simulink model "FinalProject"  (R2022a)
settings: Solver=FixedStepAuto  StartTime=0.0  StopTime=inf  FixedStep=0.1  RelTol=1e-3
model workspace (MAT data in the model file):
  SL_ROS_VariableLengthArrays_MaxSizes.CommonInfo.ArrayTruncateAction = 'EmitWarning'
  SL_ROS_VariableLengthArrays_MaxSizes.MsgTypeMap = containers.Map
  SL_ROS_VariableLengthArrays_MaxSizes.MsgTypeMap.serialization.keys = {'sensor_msgs/Image'}
  SL_ROS_VariableLengthArrays_MaxSizes.MsgTypeMap.serialization.values{1}(1).PropertyName = 'Data'
  SL_ROS_VariableLengthArrays_MaxSizes.MsgTypeMap.serialization.values{1}(1).DataType = 'uint8'
  SL_ROS_VariableLengthArrays_MaxSizes.MsgTypeMap.serialization.values{1}(1).MaxLength = 921600
  SL_ROS_VariableLengthArrays_MaxSizes.MsgTypeMap.serialization.values{1}(2).PropertyName = 'Encoding'
  SL_ROS_VariableLengthArrays_MaxSizes.MsgTypeMap.serialization.values{1}(2).DataType = 'uint8'
  SL_ROS_VariableLengthArrays_MaxSizes.MsgTypeMap.serialization.values{1}(2).MaxLength = 128
  SL_ROS_VariableLengthArrays_MaxSizes.MsgTypeMap.serialization.uniformity = 0
  SL_ROS_VariableLengthArrays_MaxSizes.MsgTypeMap.serialization.keyType = 'char'
  SL_ROS_VariableLengthArrays_MaxSizes.MsgTypeMap.serialization.valueType = 'any'
values from neighbouring files (symbols this model uses):
  WList = [0, 0, 0 ... (first row only)    [A1_WayAndObj.m]    (also in A1_WayDefAndObjSpawn.m; WList.mat = [0 6 3 9 12 15 18 0 0 6 9 0 ... (21 elements, 7x3)])
undefined symbols (not defined in the file or in its folder): Angular, gray, Linear, Rec, SDTV
libraries: robotlib x7, simulink x3, visiontextngfix x2, visionstatistics x2, visionconversions x1
settings Model: Creator=jacopo  LastModifiedBy=jacopo
settings OptimizationCC: EnhancedBackFolding=on  PassReuseOutputArgsAs=Individual arguments  ZeroExternalMemoryAtStartup=off  ZeroInternalMemoryAtStartup=off  MaxStackSize=64  OptimizeBlockOrder=speed  DifferentSizesBufferReuse=on  OptimizationCustomize=off  EfficientTunableParamExpr=on
settings DebuggingCC: ParameterTunabilityLossMsg=error
settings HardwareCC: ProdBitPerPointer=32  ProdBitPerSizeT=32  ProdBitPerPtrDiffT=32  ProdLargestAtomicFloat=None  ProdIntDivRoundTo=Undefined  ProdEndianess=Unspecified  ProdWordSize=32  ProdHWDeviceType=Generic->Unspecified (assume 32-bit Generic)
settings SFSimCC: MATLABDynamicMemAlloc=off
settings RTWCC: SystemTargetFile=ert.tlc  HardwareBoard=Robot Operating System (ROS)  TLCOptions="-aInlineSetEventsForThisBaseRateFcn=TLC_FALSE -aSuppressMultiTaskScheduler=TLC_FALSE  -aRateBasedStepFcn=0"  TemplateMakefile=ert_default_tmf  Toolchain=Catkin  TargetLang=C++
settings CodeAppCC: ForceParamTrailComments=on  IgnoreCustomStorageClasses=off  OperatorAnnotations=on  SimulinkDataObjDesc=on  SFDataObjDesc=on  InsertBlockDesc=on

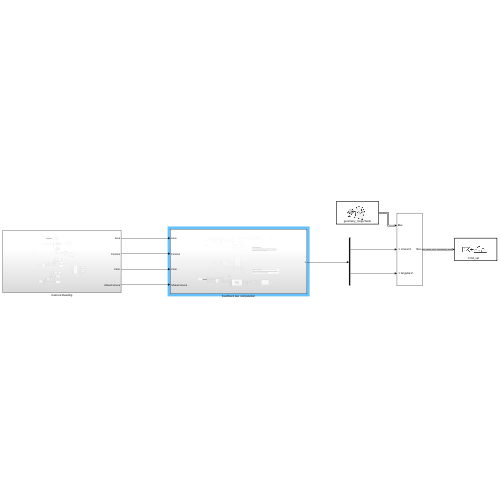
[thumbnail: Simulink's stored preview of the top-level diagram]
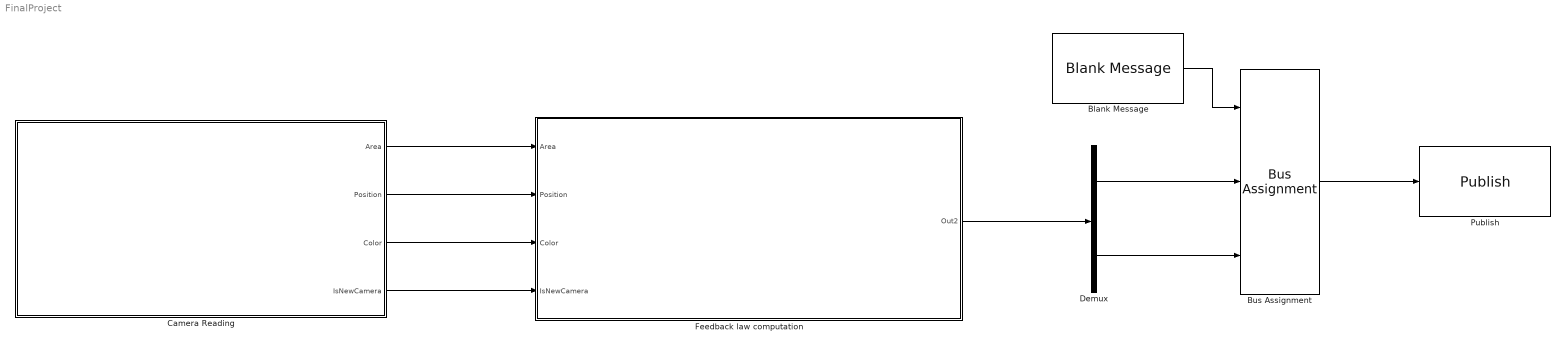
== system FinalProject ==
  Blank Message : robotlib/Blank Message  messageClass=Message  entityType=geometry_msgs/Twist  messageType=geometry_msgs/Twist  SampleTime=inf  legacyBusStruct=off
  Bus Assignment : BusAssignment  AssignedSignals=Linear.X,Angular.Z
  Camera Reading : Subsystem
  Demux : Demux  Outputs=2
  Feedback law computation : Subsystem
  Publish : robotlib/Publish  topicSource=Select from ROS network  topic=/cmd_vel  messageType=geometry_msgs/Twist  legacyBusStruct=off  messageQueueLength=1
  wires:
  Demux/1 -> Bus Assignment/2
  Blank Message/1 -> Bus Assignment/1
  Demux/2 -> Bus Assignment/3
  Bus Assignment/1 -> Publish/1
  Feedback law computation/1(Out2) -> Demux/1
  Camera Reading/4(IsNewCamera) -> Feedback law computation/4(IsNewCamera)
  Camera Reading/3(Color) -> Feedback law computation/3(Color)
  Camera Reading/2(Position) -> Feedback law computation/2(Position)
  Camera Reading/1(Area) -> Feedback law computation/1(Area)

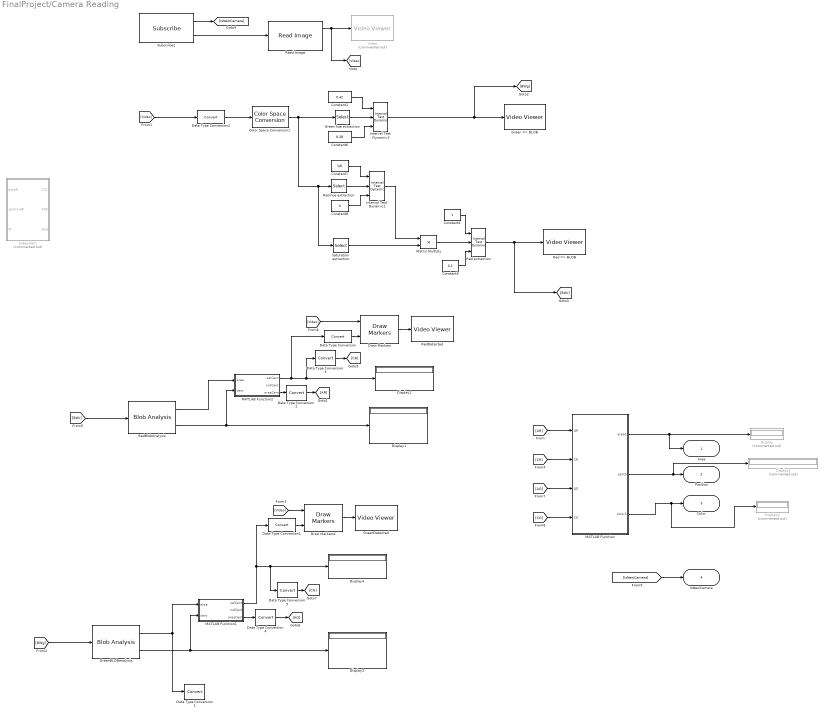
== system FinalProject/Camera Reading ==
  Color Space Conversion1 : visionconversions/Color Space  Conversion  conversion=Obsolete  conversionActive=R'G'B' to HSV  wp_str=D65  rec=Rec. 601 (SDTV)  sys=1125/60/2:1  imagePorts=One multidimensional signal
  Constant1 : Constant  Value=0.42
  Constant4 : Constant
  Constant5 : Constant  Value=0.1
  Constant6 : Constant  Value=0.28
  Constant7 : Constant  Value=1/6
  Constant8 : Constant  Value=0
  Data Type Conversion{,1,1..2,2..5} (8 alike) : DataTypeConversion  SaturateOnIntegerOverflow=off  RndMeth=Floor
  Display : Display  Commented=on
  Display{1..4} (4 alike) : Display
  Display5 : Display  Commented=on
  Display6 : Display  Commented=on
  Draw Markers : visiontextngfix/Draw Markers  shape=Star  size=30  fill=off  fillClrSource=Specify via dialog  display=User-specified value  intensity=200  color=[255 0 0]  opacity=0.6  viewport=Entire image  antialiasing=off  inType=Obsolete  imagePorts=One multidimensional signal  roundingMode=Floor  overflowMode=off  memoryMode=Specify word length  memoryWordLength=16  memoryFracLength=15  prodOutputMode=Binary point scaling  prodOutputWordLength=32  prodOutputFracLength=14
      settings: SourceProductBaseCode=VP
  Draw Markers1 : visiontextngfix/Draw Markers  shape=Plus  size=30  fill=off  fillClrSource=Specify via dialog  display=User-specified value  intensity=200  color=[255 0 0]  opacity=0.6  viewport=Entire image  antialiasing=off  inType=Obsolete  imagePorts=One multidimensional signal  roundingMode=Floor  overflowMode=off  memoryMode=Specify word length  memoryWordLength=16  memoryFracLength=15  prodOutputMode=Binary point scaling  prodOutputWordLength=32  prodOutputFracLength=14
      settings: SourceProductBaseCode=VP
  Green => BLOB : VideoViewer  colormapValue=gray(256)  FigPos=[963 1078 601 330]
  Green hue extraction : Selector  NumberOfDimensions=3  InputPortWidth=3  IndexOptions=Index vector (dialog),Index vector (dialog),Index vector (dialog)  Indices=[1:480],[1:640],1  OutputSizes=1,1,1
  GreenBLOBanalysis : visionstatistics/Blob Analysis  Tag=vipblks_row_conv  area=on  centroid=on  bBox=off  majorAxis=off  minorAxis=off  angle=off  eccentricity=off  equivDiameterSq=off  extent=off  perimeter=off  outDT=double  conn=8  isLabel=off  maxBlobs=3  warnIfNumBlobsExceeded=on  isCount=off  useMinArea=off  minArea=0  useMaxArea=off  maxArea=intmax('uint32')  excludeBorderBlob=off  isOutVarDim=off  isFill=on  fillValues=-1  roundingMode=Floor  overflowMode=off  prodOutputMode=Binary point scaling  prodOutputWordLength=32  prodOutputFracLength=16  accumMode=Binary point scaling  accumWordLength=32  accumFracLength=0  outputMode=Binary point scaling  outputWordLength=32  outputFracLength=16  firstCoeffMode=Binary point scaling  firstCoeffWordLength=16  firstCoeffFracLength=14  secondCoeffMode=Binary point scaling  secondCoeffWordLength=32  secondCoeffFracLength=16
  GreenDetected : VideoViewer  colormapValue=gray(256)  FigPos=[253 580 593 356]
  Interval Test Dynamic1 : simulink/Logic and Bit Operations/Interval Test Dynamic  IntervalClosedRight=on  IntervalClosedLeft=on  OutDataTypeStr=boolean
      settings: SourceProductBaseCode=SL
  Interval Test Dynamic3 : simulink/Logic and Bit Operations/Interval Test Dynamic  IntervalClosedRight=on  IntervalClosedLeft=on  OutDataTypeStr=boolean
      settings: SourceProductBaseCode=SL
  MATLAB Function : MATLAB Function  TreatAsAtomicUnit=on
  MATLAB Function1 : MATLAB Function  TreatAsAtomicUnit=on
  MATLAB Function2 : MATLAB Function  TreatAsAtomicUnit=on
  Matrix Multiply : Product
  Read Image : robotlib/Read Image  MaximumImageSize=[480, 640]  ImageEncoding=rgb8  ShowAlphaOutput=off  ShowErrorCodeOutput=on  VariableSizeOutputs=off
      settings: SourceProductBaseCode=RR
  Red => BLOB : VideoViewer  colormapValue=gray(256)  FigPos=[650 1078 581 344]
  Red extraction : simulink/Logic and Bit Operations/Interval Test Dynamic  IntervalClosedRight=on  IntervalClosedLeft=on  OutDataTypeStr=boolean
      settings: SourceProductBaseCode=SL
  Red hue extraction : Selector  NumberOfDimensions=3  InputPortWidth=3  IndexOptions=Index vector (dialog),Index vector (dialog),Index vector (dialog)  Indices=[1:480],[1:640],1  OutputSizes=1,1,1
  RedBlobAnalysis : visionstatistics/Blob Analysis  Tag=vipblks_row_conv  area=on  centroid=on  bBox=off  majorAxis=off  minorAxis=off  angle=off  eccentricity=off  equivDiameterSq=off  extent=off  perimeter=off  outDT=double  conn=8  isLabel=off  maxBlobs=3  warnIfNumBlobsExceeded=on  isCount=off  useMinArea=off  minArea=0  useMaxArea=off  maxArea=intmax('uint32')  excludeBorderBlob=off  isOutVarDim=off  isFill=on  fillValues=-1  roundingMode=Floor  overflowMode=off  prodOutputMode=Binary point scaling  prodOutputWordLength=32  prodOutputFracLength=16  accumMode=Binary point scaling  accumWordLength=32  accumFracLength=0  outputMode=Binary point scaling  outputWordLength=32  outputFracLength=16  firstCoeffMode=Binary point scaling  firstCoeffWordLength=16  firstCoeffFracLength=14  secondCoeffMode=Binary point scaling  secondCoeffWordLength=32  secondCoeffFracLength=16
  RedDetected : VideoViewer  colormapValue=gray(256)  FigPos=[255 1064 583 363]
  Saturation extraction : Selector  NumberOfDimensions=3  InputPortWidth=3  IndexOptions=Index vector (dialog),Index vector (dialog),Index vector (dialog)  Indices=[1:480],[1:640],2  OutputSizes=1,1,1
  Subscribe1 : robotlib/Subscribe  topicSource=Select from ROS network  topic=/camera/rgb/image_raw  messageType=sensor_msgs/Image  SampleTime=-1  legacyBusStruct=off  messageQueueLength=1
  Subsystem : Subsystem  Commented=on
  Video : VideoViewer  Commented=on  colormapValue=gray(256)  FigPos=[689 794 566 352]
  Area : Outport
  Position : Outport  Port=2
  Color : Outport  Port=3
  IsNewCamera : Outport  Port=4
  wires:
  Subscribe1/2 -> Read Image/1
  Constant7/1 -> Interval Test Dynamic1/1
  Read Image/1 -> [Video], Video/1
  Saturation extraction/1 -> Matrix Multiply/2
  Color Space Conversion1/1 -> Green hue extraction/1, Saturation extraction/1, Red hue extraction/1
  [Video] -> Data Type Conversion2/1
  Subscribe1/1 -> [IsNewCamera]
  Constant4/1 -> Red extraction/1
  Constant5/1 -> Red extraction/3
  Red hue extraction/1 -> Interval Test Dynamic1/2
  Red extraction/1 -> [BWr], Red => BLOB/1
  Matrix Multiply/1 -> Red extraction/2
  Interval Test Dynamic1/1 -> Matrix Multiply/1
  Constant8/1 -> Interval Test Dynamic1/3
  Data Type Conversion2/1 -> Color Space Conversion1/1
  Green hue extraction/1 -> Interval Test Dynamic3/2
  Constant6/1 -> Interval Test Dynamic3/3
  Constant1/1 -> Interval Test Dynamic3/1
  Interval Test Dynamic3/1 -> [BWg], Green => BLOB/1
  [BWr] -> RedBlobAnalysis/1
  RedBlobAnalysis/2 -> Display1/1, MATLAB Function2/2(cent)
  Draw Markers/1 -> RedDetected/1
  Data Type Conversion/1 -> Draw Markers/2
  [Video] -> Draw Markers/1
  RedBlobAnalysis/1 -> MATLAB Function2/1(area)
  MATLAB Function2/1(selCent) -> Data Type Conversion3/1, Display2/1, Data Type Conversion/1
  GreenBLOBanalysis/1 -> MATLAB Function1/1(area), Data Type Conversion1/1
  MATLAB Function1/1(selCent) -> Data Type Conversion1/1, Data Type Conversion5/1, Display4/1
  [Video] -> Draw Markers1/1
  Data Type Conversion1/1 -> Draw Markers1/2
  Draw Markers1/1 -> GreenDetected/1
  GreenBLOBanalysis/2 -> Display3/1, MATLAB Function1/2(cent)
  [BWg] -> GreenBLOBanalysis/1
  MATLAB Function/2(centS) -> Display5/1, Position/1
  MATLAB Function/3(colorS) -> Display6/1, Color/1
  [AR] -> MATLAB Function/1(AR)
  [CR] -> MATLAB Function/2(CR)
  [AG] -> MATLAB Function/3(AG)
  [CG] -> MATLAB Function/4(CG)
  MATLAB Function2/3(areaCent) -> Data Type Conversion2/1
  Data Type Conversion2/1 -> [AR]
  Data Type Conversion3/1 -> [CR]
  MATLAB Function1/3(areaCent) -> Data Type Conversion4/1
  Data Type Conversion4/1 -> [AG]
  Data Type Conversion5/1 -> [CG]
  MATLAB Function/1(areaS) -> Display/1, Area/1
  [IsNewCamera] -> IsNewCamera/1

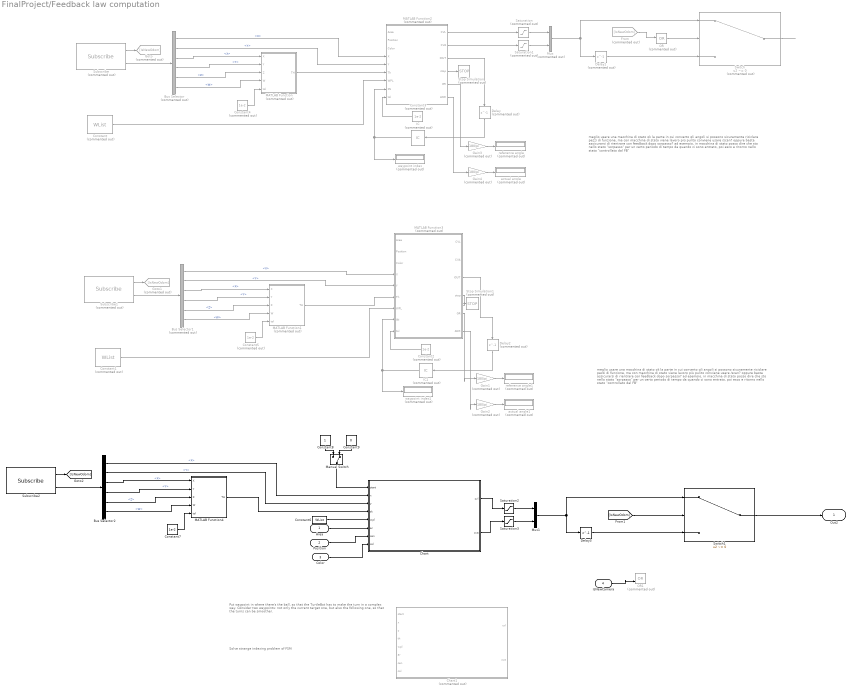
== system FinalProject/Feedback law computation ==
  note: Solve strange indexing problem of FSM
  note: Put waypoint in where there's the ball, so that the TurtleBot has to make the turn in a complex way.
      | Consider two waypoints: not only the current target one, but also the following one, so that the turns can be smoother.
  note: meglio usare una macchina di stato
      | ok la parte in cui converto gli angoli
      | si possono sicuramente riciclare pezzi di funzione, ma con macchina di stato viene lavoro più pulito
      |
      | conviene usare /scan? oppure basta assicurarsi di rientrare con feedback dopo sorpasso? ad esempio, in macchina di stato posso dire che sto nello stato "sorpasso" per un certo periodo di tempo da quando ci sono entrato, poi esco e ritorno nello stato "controllato dal FB"
  note: meglio usare una macchina di stato
      | ok la parte in cui converto gli angoli
      | si possono sicuramente riciclare pezzi di funzione, ma con macchina di stato viene lavoro più pulito
      |
      | conviene usare /scan? oppure basta assicurarsi di rientrare con feedback dopo sorpasso? ad esempio, in macchina di stato posso dire che sto nello stato "sorpasso" per un certo periodo di tempo da quando ci sono entrato, poi esco e ritorno nello stato "controllato dal FB"
  Area : Inport
  Position : Inport  Port=2
  Color : Inport  Port=3
  IsNewCamera : Inport  Port=4
  Bus Selector : BusSelector  Commented=on  OutputSignals=Pose.Pose.Position.X,Pose.Pose.Position.Y,Pose.Pose.Orientation.X,Pose.Pose.Orientation.Y,Pose.Pose.Orientation.Z,Pose.Pose.Orientation.W
  Bus Selector1 : BusSelector  Commented=on  OutputSignals=Pose.Pose.Position.X,Pose.Pose.Position.Y,Pose.Pose.Orientation.X,Pose.Pose.Orientation.Y,Pose.Pose.Orientation.Z,Pose.Pose.Orientation.W
  Bus Selector2 : BusSelector  OutputSignals=Pose.Pose.Position.X,Pose.Pose.Position.Y,Pose.Pose.Orientation.X,Pose.Pose.Orientation.Y,Pose.Pose.Orientation.Z,Pose.Pose.Orientation.W
  Chart : Stateflow chart  TreatAsAtomicUnit=on
  Chart1 : Stateflow chart  Commented=on  TreatAsAtomicUnit=on
  Constant : Constant  Commented=on  Value=WList
  Constant1 : Constant  Commented=on  Value=WList
  Constant{2..5} (4 alike) : Constant  Commented=on  Value=1e-2
  Constant6 : Constant  Value=WList
  Constant7 : Constant  Value=1e-2
  Constant8 : Constant
  Constant9 : Constant  Value=0
  Delay : Delay  Commented=on  DelayLength=1
  Delay1 : Delay  Commented=on  DelayLength=1
  Delay2 : Delay  Commented=on  DelayLength=1
  Delay3 : Delay  DelayLength=1
  From : From  Commented=on  GotoTag=IsNewOdom
  Gain{1..4} (4 alike) : Gain  Commented=on  Gain=180/pi
  Goto : Goto  Commented=on  GotoTag=IsNewOdom
  Goto1 : Goto  Commented=on  GotoTag=IsNewOdom
  IC : InitialCondition  Commented=on
  IC1 : InitialCondition  Commented=on
  MATLAB Function : MATLAB Function  Commented=on  TreatAsAtomicUnit=on
  MATLAB Function1 : MATLAB Function  Commented=on  TreatAsAtomicUnit=on
  MATLAB Function2 : MATLAB Function  Commented=on  TreatAsAtomicUnit=on
  MATLAB Function3 : MATLAB Function  Commented=on  TreatAsAtomicUnit=on
  MATLAB Function4 : MATLAB Function  TreatAsAtomicUnit=on
  Manual Switch : ManualSwitch  CurrentSetting=0
  Mux : Mux  Commented=on  Inputs=2
  Mux1 : Mux  Inputs=2
  OR : Logic  Commented=on  Operator=OR  IconShape=distinctive  AllPortsSameDT=off  OutDataTypeStr=boolean
  OR1 : Logic  Commented=on  Operator=OR  IconShape=distinctive  AllPortsSameDT=off  OutDataTypeStr=boolean
  Saturation : Saturate  Commented=on  UpperLimit=0.2  LowerLimit=-0.2
  Saturation1 : Saturate  Commented=on  UpperLimit=0.4  LowerLimit=-0.4
  Saturation2 : Saturate  UpperLimit=0.2  LowerLimit=-0.2
  Saturation3 : Saturate  UpperLimit=0.4  LowerLimit=-0.4
  Stop Simulation : Stop  Commented=on
  Stop Simulation1 : Stop  Commented=on
  Subscribe : robotlib/Subscribe  Commented=on  topicSource=Select from ROS network  topic=/odom  messageType=nav_msgs/Odometry  SampleTime=-1  legacyBusStruct=off  messageQueueLength=1
  Subscribe1 : robotlib/Subscribe  Commented=on  topicSource=Select from ROS network  topic=/odom  messageType=nav_msgs/Odometry  SampleTime=-1  legacyBusStruct=off  messageQueueLength=1
  Subscribe2 : robotlib/Subscribe  topicSource=Select from ROS network  topic=/odom  messageType=nav_msgs/Odometry  SampleTime=-1  legacyBusStruct=off  messageQueueLength=1
  Switch : Switch  Commented=on  Criteria=u2 ~= 0  SaturateOnIntegerOverflow=off  InputSameDT=off
  Switch1 : Switch  Criteria=u2 ~= 0  SaturateOnIntegerOverflow=off  InputSameDT=off
  actual angle : Display  Commented=on
  actual angle1 : Display  Commented=on
  reference angle : Display  Commented=on
  reference angle1 : Display  Commented=on
  waypoint index : Display  Commented=on
  waypoint index1 : Display  Commented=on
  Out2 : Outport
  wires:
  Delay/1 -> IC/1
  IC/1 -> MATLAB Function2/8(IIN), waypoint index/1
  Constant/1 -> MATLAB Function2/7(WPL)
  Constant3/1 -> MATLAB Function2/9(tol)
  Bus Selector/6 -> MATLAB Function/4(W)  "<W>"
  Gain4/1 -> actual angle/1
  MATLAB Function2/4(stop) -> Stop Simulation/1
  Bus Selector/5 -> MATLAB Function/3(Z)  "<Z>"
  MATLAB Function2/6(ANG) -> Gain4/1
  Bus Selector/3 -> MATLAB Function/1(X)  "<X>"
  Saturation/1 -> Mux/1
  MATLAB Function/1(TH) -> MATLAB Function2/6(Th)
  MATLAB Function2/5(GR) -> Gain3/1
  Gain3/1 -> reference angle/1
  MATLAB Function2/2(CVA) -> Saturation1/1
  MATLAB Function2/1(CVL) -> Saturation/1
  MATLAB Function2/3(IOUT) -> Delay/1
  Subscribe/1 -> Goto/1
  Subscribe/2 -> Bus Selector/1
  Constant4/1 -> MATLAB Function/5(tol)
  Bus Selector/2 -> MATLAB Function2/5(Y)  "<Y>"
  Bus Selector/1 -> MATLAB Function2/4(X)  "<X>"
  Saturation1/1 -> Mux/2
  Bus Selector/4 -> MATLAB Function/2(Y)  "<Y>"
  From/1 -> OR/1
  Delay1/1 -> Switch/3
  Mux/1 -> Switch/1, Delay1/1
  Switch/1 -> ?
  OR/1 -> Switch/2
  ? -> OR/2
  MATLAB Function3/3(IOUT) -> Delay2/1
  Bus Selector1/1 -> MATLAB Function3/4(X)  "<X>"
  Constant2/1 -> MATLAB Function3/9(tol)
  Gain2/1 -> actual angle1/1
  MATLAB Function3/5(GR) -> Gain1/1
  IC1/1 -> MATLAB Function3/8(IIN), waypoint index1/1
  Gain1/1 -> reference angle1/1
  Constant1/1 -> MATLAB Function3/7(WPL)
  MATLAB Function3/6(ANG) -> Gain2/1
  Bus Selector1/6 -> MATLAB Function1/4(W)  "<W>"
  MATLAB Function3/4(stop) -> Stop Simulation1/1
  MATLAB Function1/1(TH) -> MATLAB Function3/6(Th)
  Bus Selector1/5 -> MATLAB Function1/3(Z)  "<Z>"
  Subscribe1/2 -> Bus Selector1/1
  Bus Selector1/2 -> MATLAB Function3/5(Y)  "<Y>"
  Subscribe1/1 -> Goto1/1
  Delay2/1 -> IC1/1
  Constant5/1 -> MATLAB Function1/5(tol)
  Bus Selector1/3 -> MATLAB Function1/1(X)  "<X>"
  Bus Selector1/4 -> MATLAB Function1/2(Y)  "<Y>"
  Color/1 -> Chart/8(col)
  Position/1 -> Chart/7(cen)
  Area/1 -> Chart/6(ar)
  Constant6/1 -> Chart/5(wpl)
  Bus Selector2/1 -> Chart/2(x)  "<X>"
  Constant7/1 -> MATLAB Function4/5(tol)
  Bus Selector2/6 -> MATLAB Function4/4(W)  "<W>"
  MATLAB Function4/1(TH) -> Chart/4(th)
  Bus Selector2/5 -> MATLAB Function4/3(Z)  "<Z>"
  Subscribe2/1 -> [IsNewOdom]
  Bus Selector2/3 -> MATLAB Function4/1(X)  "<X>"
  Subscribe2/2 -> Bus Selector2/1
  Bus Selector2/2 -> Chart/3(y)  "<Y>"
  Bus Selector2/4 -> MATLAB Function4/2(Y)  "<Y>"
  Manual Switch/1 -> Chart/1(start)
  Constant8/1 -> Manual Switch/1
  Constant9/1 -> Manual Switch/2
  Saturation2/1 -> Mux1/1
  Switch1/1 -> Out2/1
  Chart/2(cva) -> Saturation3/1
  Chart/1(cvl) -> Saturation2/1
  [IsNewOdom] -> Switch1/2
  IsNewCamera/1 -> OR1/2
  Saturation3/1 -> Mux1/2
  Mux1/1 -> Switch1/1, Delay3/1
  Delay3/1 -> Switch1/3

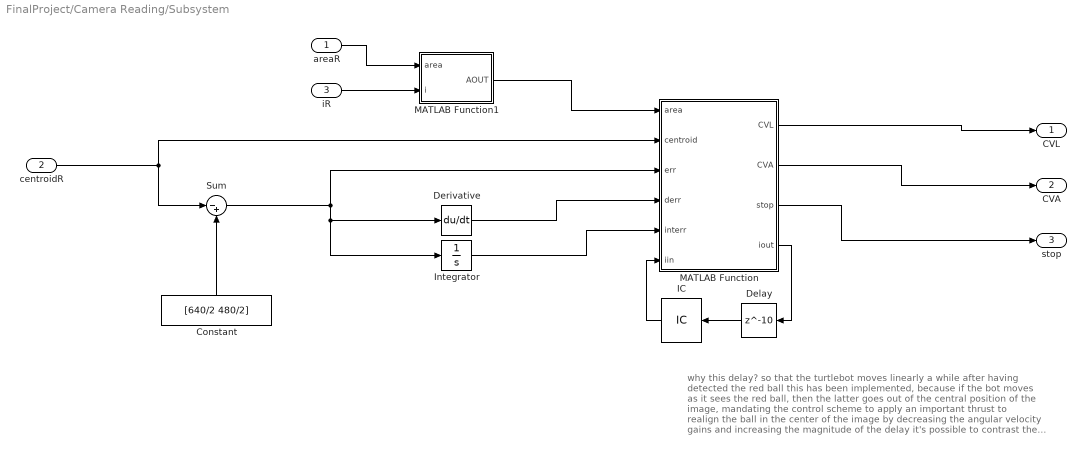
== system FinalProject/Camera Reading/Subsystem ==
  note: why this delay? so that the turtlebot moves linearly a while after
      | having detected the red ball
      | this has been implemented, because if the bot moves as it sees
      | the red ball, then the latter goes out of the central position of the image,
      | mandating the control scheme to apply an important thrust to realign
      | the ball in the center of the image
      | by decreasing the angular velocity gains and increasing the magnitude
      | of the delay it's possible to contrast the wobbly motion, caused by
      | a synergic cooperation of high gains and moving linearly too early
  areaR : Inport
  centroidR : Inport  Port=2
  iR : Inport  Port=3
  Constant : Constant  Value=[640/2 480/2]  VectorParams1D=off
  Delay : Delay  DelayLength=10
  Derivative : Derivative
  IC : InitialCondition  Value=0
  Integrator : Integrator
  MATLAB Function : MATLAB Function  TreatAsAtomicUnit=on
  MATLAB Function1 : MATLAB Function  TreatAsAtomicUnit=on
  Sum : Sum  Inputs=|-+
  CVL : Outport
  CVA : Outport  Port=2
  stop : Outport  Port=3
  wires:
  MATLAB Function/3(stop) -> stop/1
  areaR/1 -> MATLAB Function1/1(area)
  MATLAB Function/2(CVA) -> CVA/1
  MATLAB Function/1(CVL) -> CVL/1
  MATLAB Function1/1(AOUT) -> MATLAB Function/1(area)
  iR/1 -> MATLAB Function1/2(i)
  centroidR/1 -> Sum/1, MATLAB Function/2(centroid)
  Constant/1 -> Sum/2
  Sum/1 -> Integrator/1, Derivative/1, MATLAB Function/3(err)
  Derivative/1 -> MATLAB Function/4(derr)
  Integrator/1 -> MATLAB Function/5(interr)
  Delay/1 -> IC/1
  MATLAB Function/4(iout) -> Delay/1
  IC/1 -> MATLAB Function/6(iin)

== matlab function FinalProject/Camera Reading/Subsystem/MATLAB Function ==
  data: area input; CVL output; centroid input; CVA output; err input; stop output; derr input; interr input; iin input; iout output
function [CVL, CVA, stop, iout] = fcn(area, centroid, err, derr, interr, iin)

NC = 2; % max number of centroids
NoCV = - ones(NC, 2);

if centroid == NoCV
    CVL = 0;
    CVA = 0.2;
    iout = 0; %add
else
    iout = 1; %add
    kPL = 0.05;
%     kPA = 0.1;
%     kPA = 0.01;
    kPA = 0.003; % 0.01 is too high % 0.005 mmmh almost
    kDA = 0.01*0;
    kIA = 0;
    
    ERR = err(1);
    dERR = derr(1);
    intERR = interr(1);

    if iin == 1  %add
        CVL = kPL*area;
    else
        CVL = 0;
    end

    CVA = kPA*ERR + kDA*dERR + kIA*intERR;
end

maxA = 0.9*(640*480);

if area < maxA
    stop = 0;
else
    CVL = 0;
    CVA = 0;
    stop = 1;
end


% % centroidsel = centroid( centroid ~= [-1 -1])'; % not that robust

== matlab function FinalProject/Camera Reading/MATLAB Function2 ==
  data: area input; cent input; selCent output; indCent output; areaCent output
function [selCent, indCent, areaCent]  = fcn(area,cent)

[areaCent, indCent] = max(area);

if ~isempty(indCent)
    selCent = cent(indCent,:);
else 
    selCent = [0,0];
end

== matlab function FinalProject/Camera Reading/Subsystem/MATLAB Function1 ==
  data: area input; AOUT output; i input
function AOUT = fcn(area, i)

AOUT = area(i, 1);

== matlab function FinalProject/Camera Reading/MATLAB Function ==
  data: AR input; CR input; areaS output; centS output; colorS output; AG input; CG input
function [areaS, centS, colorS] = fcn(AR, CR, AG, CG)

% 1 is red, 2 is green, 0 is none

if AR > AG
    areaS = AR;
    centS = CR;
    colorS = 1;
elseif AR < AG
    areaS = AG;
    centS = CG;
    colorS = 2;
else
    areaS = 0;
    centS = [0 0];
    colorS = 0;
end

== matlab function FinalProject/Feedback law computation/MATLAB Function ==
  data: X input; TH output; Y input; Z input; W input; tol input
function TH = fromQuat2Eu(X, Y, Z, W, tol)



ANGLE = quat2eul([W, X, Y, Z]);

TH = ANGLE(1);

== matlab function FinalProject/Feedback law computation/MATLAB Function2 ==
  data: Area input; Position input; Color input; X input; CVL output; Y input; Th input; WPL input; CVA output; IOUT output; IIN input; stop output; tol input; GR output; ANG output
function [CVL, CVA, IOUT, stop, GR, ANG] = FBRegulator(Area, Position, Color, X, Y, Th, WPL, IIN, tol)

% kPL = 1;
kPA = 2; %0.8 %1.2

POSr = WPL(IIN, :);

Xr = POSr(1); Yr = POSr(2); Thr = POSr(3);

if pi < Thr && Thr < 2*pi
    Thr = Thr - 2*pi;
end

Gr = Thr;

Z = (Xr - X) + 1i*(Yr - Y);

dist = abs(Z);

% if dist <= 0.2
%     kPL = 0.4;
% end

if dist <= 0.1

    if (Th > tol) && (- pi + tol < Gr && Gr < - pi/2 - tol) % Gr < - tol
        Gr = Gr + 2*pi;
    elseif (- pi + tol < Th && Th < - pi/2 - tol) && (Gr > tol)
        Th = Th + 2*pi;
    end
    
else

    Gr = angle(Z);

    if (Th > tol) && (- pi + tol < Gr && Gr < - pi/2 - tol) % Gr < - tol
        Gr = Gr + 2*pi;
    elseif (- pi + tol < Th && Th < - pi/2 - tol) && (Gr > tol)
        Th = Th + 2*pi;
    end

end

errTh = Gr - Th;
GR = Gr;

ANG = Th;

% CVL = kPL*dist;
% CVL = kPL*0.1;
% CVL = kPL*0.2; % faster attempt
% CVL = 0.45*dist; %0.8 original, %0.4 not robust
% CVA = kPA*errTh;


if dist <= 0.05 
   stop = 0;
   CVL = 0;
   CVA = kPA*errTh;
   if abs(errTh) <= 0.05
        IOUT = IIN + 1;
        if IIN == 6
            CVA = 0;
            stop = 1;
        end
   else
       IOUT = IIN;
   end
else
    if Area > 0.2*(480*640)
        if Color == 1
            CVL = 0.15;
            CVA = 0.3;
        elseif Color == 2
            CVL = 0.15;
            CVA = -0.3;
        else
            CVA = 0.1;
            CVL = 0.1;
        end
%        a variable can be outputted with a delay, to make sure we will
%        not exit the overtake phase
    else
        CVL = 0.1*dist;
        CVA = kPA*errTh;
    end
%     CVA = kPA*errTh;
    IOUT = IIN;
    stop = 0;
end

== matlab function FinalProject/Feedback law computation/MATLAB Function1 ==
  data: X input; TH output; Y input; Z input; W input; tol input
function TH = fromQuat2Eu(X, Y, Z, W, tol)



ANGLE = quat2eul([W, X, Y, Z]);

TH = ANGLE(1);

== matlab function FinalProject/Feedback law computation/MATLAB Function3 ==
  data: Area input; Position input; Color input; X input; CVL output; Y input; Th input; WPL input; CVA output; IOUT output; IIN input; stop output; tol input; GR output; ANG output
function [CVL, CVA, IOUT, stop, GR, ANG] = FBRegulator(Area, Position, Color, X, Y, Th, WPL, IIN, tol)

% kPL = 1;
kPA = 2; %0.8 %1.2

POSr = WPL(IIN, :);

Xr = POSr(1); Yr = POSr(2); Thr = POSr(3);

if pi < Thr && Thr < 2*pi
    Thr = Thr - 2*pi;
end

Gr = Thr;

Z = (Xr - X) + 1i*(Yr - Y);

dist = abs(Z);

% if dist <= 0.2
%     kPL = 0.4;
% end

if dist <= 0.1

    if (Th > tol) && (- pi + tol < Gr && Gr < - pi/2 - tol) % Gr < - tol
        Gr = Gr + 2*pi;
    elseif (- pi + tol < Th && Th < - pi/2 - tol) && (Gr > tol)
        Th = Th + 2*pi;
    end
    
else

    Gr = angle(Z);

    if (Th > tol) && (- pi + tol < Gr && Gr < - pi/2 - tol) % Gr < - tol
        Gr = Gr + 2*pi;
    elseif (- pi + tol < Th && Th < - pi/2 - tol) && (Gr > tol)
        Th = Th + 2*pi;
    end

end

errTh = Gr - Th;
GR = Gr;

ANG = Th;

% CVL = kPL*dist;
% CVL = kPL*0.1;
% CVL = kPL*0.2; % faster attempt
% CVL = 0.45*dist; %0.8 original, %0.4 not robust
% CVA = kPA*errTh;


if dist <= 0.05 
   stop = 0;
   CVL = 0;
   CVA = kPA*errTh;
   if abs(errTh) <= 0.05
        IOUT = IIN + 1;
        if IIN == 6
            CVA = 0;
            stop = 1;
        end
   else
       IOUT = IIN;
   end
else
    if Area > 0.2*(480*640)
        if Color == 1
            CVL = 0.15;
            CVA = 0.3;
        elseif Color == 2
            CVL = 0.15;
            CVA = -0.3;
        else
            CVA = 0.1;
            CVL = 0.1;
        end
%        a variable can be outputted with a delay, to make sure we will
%        not exit the overtake phase
    else
        CVL = 0.1*dist;
        CVA = kPA*errTh;
    end
%     CVA = kPA*errTh;
    IOUT = IIN;
    stop = 0;
end

== stateflow chart FinalProject/Feedback law computation/Chart ==
  state RedOvertaking
    [cvl, cva, overT, aDec] = overtakingR(cvl, cva, overT);
  state FBMotion
    [Dist, ErrTh] = disterrfun(x, y, th, wpl, index)
    cvl = kPL*Dist;
    cva = kPA*ErrTh;
  state Still
    cvl = 0;
    cva = 0;
    index = 1;
    kPL = 0.48;
    kPA = 2;
    overT = 0;
  state GreenOvertaking
    [cvl, cva, overT, aDec] = overtakingG(cvl, cva, overT);
  state Turning
    [Dist, ErrTh] = disterrfun(x, y, th, wpl, index)
    cvl = 0;
    cva = (0.9*kPA)*ErrTh;
  RedOvertaking -> RedOvertaking [order 2] : [aDec == 1]
  FBMotion -> RedOvertaking [order 1] : [ar > 0.1*(480*640) && col == 1 ] {aDec = 1}
  RedOvertaking -> FBMotion [order 1] : [aDec == 0] {overT = 1}
  FBMotion -> FBMotion [order 5] : [Dist > 0.05]
  FBMotion -> GreenOvertaking [order 4] : [ar > 0.1*(480*640) && col == 2] {aDec = 1}
  Still -> FBMotion [order 2] : [start == 1]
  (default) -> Still
  FBMotion -> Still [order 3] : [index == 6]
  Still -> Still [order 1] : [start == 0]
  Turning -> FBMotion [order 2] : [abs(ErrTh) <= 0.05] {index = index + 1}
  FBMotion -> Turning [order 2] : [Dist <= 0.05 ]
  GreenOvertaking -> FBMotion [order 2] : [aDec == 0] {overT = 1}
  GreenOvertaking -> GreenOvertaking [order 1] : [aDec == 1]
  Turning -> Turning [order 1] : [abs(ErrTh) > 0.05]
  data: X function_input; Y function_input; Th function_input; WPL function_input; dist function_output; errTh function_output; IND function_input; CVL function_output; CVA function_output; CVLin function_input; CVAin function_input; overt function_output; overt function_input; adec function_output; CVL function_output; CVA function_output; CVLin function_input; CVAin function_input; overt function_output; overt function_input; adec function_output; start input; x input; y input; th input; wpl input; ar input; cen input; col input; Dist local; ErrTh local; cvl output; cva output; index local; kPA local; kPL local; aDec local; overT local
  function [dist, errTh] = disterrfun(X, Y, Th, WPL, IND):
    | function [dist, errTh] = disterrfun(X, Y, Th, WPL, IND)
    |  
    | tol = 1e-2;
    | 
    | POSr = WPL(IND, :);
    | 
    | Xr = POSr(1); Yr = POSr(2); Thr = POSr(3);
    | 
    | if pi < Thr && Thr < 2*pi
    |     Thr = Thr - 2*pi;
    | end
    | 
    | Gr = Thr;
    | Z = (Xr - X) + 1i*(Yr - Y);
    | dist = abs(Z);
    | 
    | 
    | if dist <= 0.1
    |     if (Th > tol) && (- pi + tol < Gr && Gr < - pi/2 - tol) % Gr < - tol
    |         Gr = Gr + 2*pi;
    |     elseif (- pi + tol < Th && Th < - pi/2 - tol) && (Gr > tol)
    |         Th = Th + 2*pi;
    |     end
    | else
    |     Gr = angle(Z);
    |     if (Th > tol) && (- pi + tol < Gr && Gr < - pi/2 - tol) % Gr < - tol
    |         Gr = Gr + 2*pi;
    |     elseif (- pi + tol < Th && Th < - pi/2 - tol) && (Gr > tol)
    |         Th = Th + 2*pi;
    |     end
    | end
    | 
    | errTh = Gr - Th;
  function [CVL, CVA, overt, adec] = overtakingR(CVLin, CVAin, overt):
    | function [CVL, CVA, overt, adec] = overtakingR(CVLin, CVAin, overt)
    | 
    | CVL = CVLin;
    | tTurn = 40; %35;
    | tStop = 75; %70;
    | % tStop = 90;
    | 
    | % turnVel = 0.2;
    | 
    | vR = 0.1;
    | wR = 0.1;
    | 
    | % v = min(0.2, max(-0.2, CVL)); % it simulates saturation
    | 
    | v = CVL*(CVL <= 0.2) + 0.2*(CVL > 0.2);
    | 
    | turnVel = wR*v/vR;
    | 
    | if overt < tTurn
    |     CVA = turnVel;
    |     adec = 1;
    | elseif tTurn < overt && overt < tStop
    |     CVA = 0;
    |     adec = 1;
    | else
    |     CVA = CVAin;
    |     adec = 0;
    | end
    | 
    | overt = overt + 1;
  function [CVL, CVA, overt, adec] = overtakingG(CVLin, CVAin, overt):
    | function [CVL, CVA, overt, adec] = overtakingG(CVLin, CVAin, overt)
    | 
    | CVL = CVLin;
    | tTurn = 40; %35;
    | tStop = 75; %70;
    | % tStop = 90;
    | 
    | % turnVel = 0.2;
    | 
    | vR = 0.1;
    | wR = 0.1;
    | 
    | % v = min(0.2, max(-0.2, CVL)); % it simulates saturation
    | 
    | v = CVL*(CVL <= 0.2) + 0.2*(CVL > 0.2);
    | 
    | turnVel = wR*v/vR;
    | 
    | if overt < tTurn
    |     CVA = -turnVel;
    |     adec = 1;
    | elseif tTurn < overt && overt < tStop
    |     CVA = 0;
    |     adec = 1;
    | else
    |     CVA = CVAin;
    |     adec = 0;
    | end
    | 
    | overt = overt + 1;
    | 
    | % wobbling perché riconosce altro colore!

== matlab function FinalProject/Feedback law computation/MATLAB Function4 ==
  data: X input; TH output; Y input; Z input; W input; tol input
function TH = fromQuat2Eu(X, Y, Z, W, tol)



ANGLE = quat2eul([W, X, Y, Z]);

TH = ANGLE(1);

== stateflow chart FinalProject/Feedback law computation/Chart1 ==
  state FBMotion
    [Dist, ErrTh] = disterrfun(x, y, th, wpl, index)
    cvl = kPL*Dist;
    cva = kPA*ErrTh;
  state Still
    cvl = 0;
    cva = 0;
    index = 1;
    kPL = 0.48;
    kPA = 2;
    overT = 0;
  state Overtaking
    [cvl, cva, overT, aDec] = overtaking(ar, cen, col, cvl, cva, overT);
  state Turning
    [Dist, ErrTh] = disterrfun(x, y, th, wpl, index)
    cvl = 0;
    cva = kPA*ErrTh;
  FBMotion -> FBMotion [order 4] : [Dist > 0.05 ]
  Still -> FBMotion [order 2] : [start == 1]
  (default) -> Still
  FBMotion -> Overtaking [order 1] : [ar > 0.1*(480*640)] {aDec = 1}
  FBMotion -> Still [order 3] : [index == 6]
  Overtaking -> FBMotion [order 1] : [aDec == 0] {overT = 1}
  Still -> Still [order 1] : [start == 0]
  Turning -> FBMotion [order 2] : [abs(ErrTh) <= 0.05] {index = index + 1}
  FBMotion -> Turning [order 2] : [Dist <= 0.05 ]
  Overtaking -> Overtaking [order 2] : [aDec == 1]
  Turning -> Turning [order 1] : [abs(ErrTh) > 0.05]
  data: X function_input; Y function_input; Th function_input; WPL function_input; dist function_output; errTh function_output; IND function_input; Ar function_input; Cen function_input; Col function_input; CVL function_output; CVA function_output; CVLin function_input; CVAin function_input; overt function_output; overt function_input; adec function_output; start input; x input; y input; th input; wpl input; ar input; cen input; col input; Dist local; ErrTh local; cvl output; cva output; index local; kPA local; kPL local; aDec local; overT local
  function [dist, errTh] = disterrfun(X, Y, Th, WPL, IND):
    | function [dist, errTh] = disterrfun(X, Y, Th, WPL, IND)
    |  
    | tol = 1e-2;
    | 
    | POSr = WPL(IND, :);
    | 
    | Xr = POSr(1); Yr = POSr(2); Thr = POSr(3);
    | 
    | if pi < Thr && Thr < 2*pi
    |     Thr = Thr - 2*pi;
    | end
    | 
    | Gr = Thr;
    | Z = (Xr - X) + 1i*(Yr - Y);
    | dist = abs(Z);
    | 
    | 
    | if dist <= 0.1
    |     if (Th > tol) && (- pi + tol < Gr && Gr < - pi/2 - tol) % Gr < - tol
    |         Gr = Gr + 2*pi;
    |     elseif (- pi + tol < Th && Th < - pi/2 - tol) && (Gr > tol)
    |         Th = Th + 2*pi;
    |     end
    | else
    |     Gr = angle(Z);
    |     if (Th > tol) && (- pi + tol < Gr && Gr < - pi/2 - tol) % Gr < - tol
    |         Gr = Gr + 2*pi;
    |     elseif (- pi + tol < Th && Th < - pi/2 - tol) && (Gr > tol)
    |         Th = Th + 2*pi;
    |     end
    | end
    | 
    | errTh = Gr - Th;
  function [CVL, CVA, overt, adec] = overtaking(Ar, Cen, Col, CVLin, CVAin, overt):
    | function [CVL, CVA, overt, adec] = overtaking(Ar, Cen, Col, CVLin, CVAin, overt)
    | 
    | CVL = CVLin;
    | tTurn = 60;
    | tStop = 90;
    | 
    | % turnVel = 0.2;
    | 
    | vR = 0.2;
    | wR = 0.4;
    | 
    | % v = min(0.2, max(-0.2, CVL)); % it simulates saturation
    | 
    | v = CVL*(CVL <= 0.2) + 0.2*(CVL > 0.2);
    | 
    | turnVel = wR*v/vR;
    | 
    | if overt < tTurn
    |     if Col == 1
    |         CVA = turnVel;
    |     elseif Col == 2
    |         CVA = -turnVel;
    |     else
    |         CVA = CVAin;
    |     end
    |     adec = 1;
    | elseif tTurn < overt && overt < tStop
    |     CVA = 0;
    |     adec = 1;
    | else
    |     CVA = CVAin;
    |     adec = 0;
    | end
    | 
    | overt = overt + 1;
    | 
    | % wobbling perché riconosce altro colore!

== matlab function FinalProject/Camera Reading/MATLAB Function1 ==
  data: area input; cent input; selCent output; indCent output; areaCent output
function [selCent, indCent, areaCent]  = fcn(area,cent)

[areaCent, indCent] = max(area);

if ~isempty(indCent)
    selCent = cent(indCent,:);
else 
    selCent = [0,0];
end
